simulink model "serial_receive"  (R2016a)
settings: Solver=FixedStepAuto  StartTime=0.0  StopTime=inf  FixedStep=0.01  RelTol=1e-3
undefined symbols (not defined in the file): serial
libraries: instrumentlib x3, aerolibanimutils x1
settings Model: Creator=lsr  LastModifiedBy=lsr

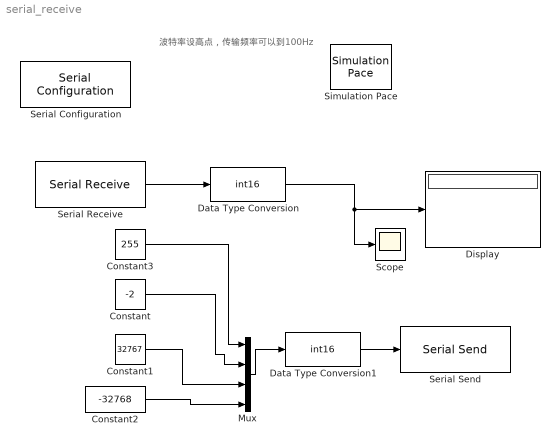
== system serial_receive ==
  note: 波特率设高点，传输频率可以到100Hz
  Constant : Constant  Value=-2
  Constant1 : Constant  Value=32767
  Constant2 : Constant  Value=-32768
  Constant3 : Constant  Value=255
  Data Type Conversion : DataTypeConversion  OutDataTypeStr=int16
  Data Type Conversion1 : DataTypeConversion  OutDataTypeStr=int16
  Display : Display
  Mux : Mux
  Scope : Scope
  Serial Configuration : instrumentlib/Serial Configuration  Priority=-200000  ComPortMenu=COM15  ComPort=COM15  ObjConstructor=serial('COM15');  BaudRate=9600  DataBits=8  Parity=none  StopBits=1  FlowControl=none  Timeout=0.01  ByteOrder=BigEndian
  Serial Receive : instrumentlib/Serial Receive  ComPortMenu=<Please select a port...>  ComPort=COM15  ObjConstructor=serial('COM15');  Terminator=<none>  DataSize="[1  3]"  DataType=int16  EnableBlockingMode=on  ActionDataUnavailable=Output custom value  CustomValue=0  SampleTime=0.01
  Serial Send : instrumentlib/Serial Send  ComPortMenu=<Please select a port...>  ComPort=COM15  ObjConstructor=serial('COM15');  Terminator=<none>  EnableBlockingMode=on
  Simulation Pace : aerolibanimutils/Simulation Pace  SimulationPace=1  SleepMode=MATLAB Thread  OutputPaceError=off  SampleTime=0.01
  wires:
  Data Type Conversion/1 -> Scope/1, Display/1
  Mux/1 -> Data Type Conversion1/1
  Constant/1 -> Mux/2
  Data Type Conversion1/1 -> Serial Send/1
  Constant1/1 -> Mux/3
  Constant3/1 -> Mux/1
  Constant2/1 -> Mux/4
  Serial Receive/1 -> Data Type Conversion/1
